simulink model "plant"  (R2020a)
settings: Solver=VariableStepAuto  StartTime=0.0  StopTime=20.0  RelTol=1e-3
values from neighbouring files (symbols this model uses):
  Ts = 0.1    [main_adaptive_mpc.m]
libraries: sharedtransform x1, shared6dof x1, mpclib x1
settings Model: Creator=Lamarre  LastModifiedBy=Lamarre

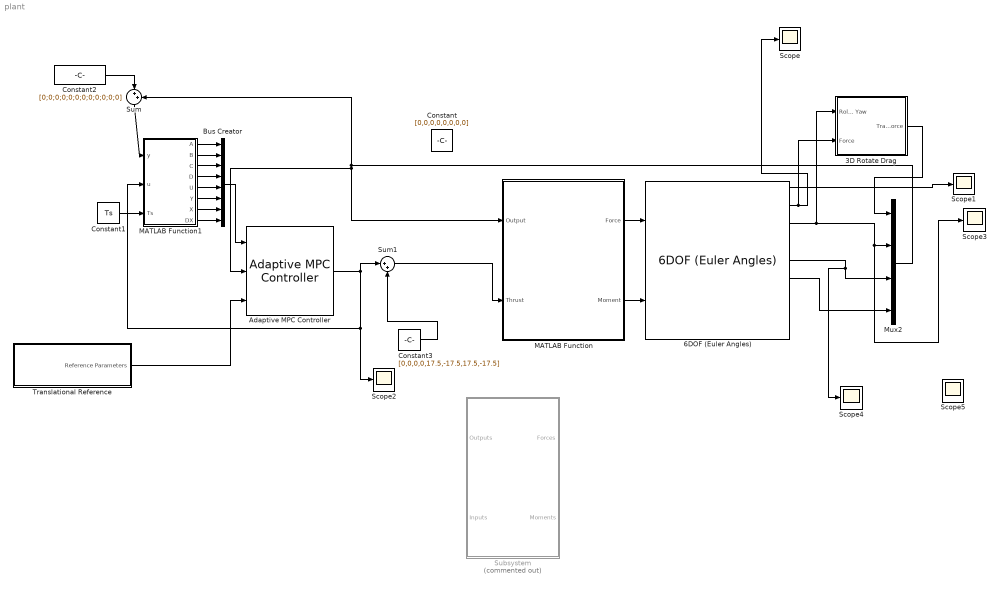
== system plant ==
  3D Rotate Drag : Subsystem
  6DOF (Euler Angles) : shared6dof/6DOF (Euler Angles)  units=Metric (MKS)  mtype=Fixed  rep=Euler Angles  xme_0=[0 0 0]  Vm_0=[0 0 0]  eul_0=[0 0 0]  pm_0=[0 0 0]  mass_0=mass  mass_e=0.5  mass_f=2.0  inertia=I  inertia_e=eye(3)  inertia_f=2*eye(3)  k_quat=1.0  vre_flag=on  abi_flag=on  aMode=0  xme_statename=''  Vm_statename=''  eul_statename=''  quat_statename=''  pm_statename=''  mass_statename=''
      settings: SourceProductBaseCode=AE,PW,MT,VE,VP
  Adaptive MPC Controller : mpclib/Adaptive MPC Controller  SCDEnableBlockLinearizationSpecification=on  mpcobj=mpcobj  enable_value=0  updateMPCinCallerWorkspace=on  md_inport=off  mv_inport=off  uref_inport=off  return_cost=off  return_mvseq=off  return_qpstatus=off  return_xseq=off  return_state=off  return_ovseq=off  state_inport=off  isltv_plant=off  umin_inport=off  umax_inport=off  ymin_inport=off  ymax_inport=off  cc_inport=off  ywt_inport=off  uwt_inport=off  duwt_inport=off  rhoeps_inport=off  pm_inport=off  MaximumP=10  HorizonChoice=FixedHorizon  BlockDataType=double  SampleTimeInherited=off  switch_inport=off
  Bus Creator : BusCreator  Inputs=8
  Constant : Constant  Value=[0,0,0,0,0,0,0,0]
  Constant1 : Constant  Value=Ts
  Constant2 : Constant  Value=[0;0;0;0;0;0;0;0;0;0;0;0]  VectorParams1D=off
  Constant3 : Constant  Value=[0,0,0,0,17.5,-17.5,17.5,-17.5]
  MATLAB Function : MATLAB Function  TreatAsAtomicUnit=on
  MATLAB Function1 : MATLAB Function  TreatAsAtomicUnit=on
  Mux2 : Mux
  Scope{,1..5} (6 alike) : Scope
  Subsystem : Subsystem  Commented=on
  Sum : Sum  Inputs=|++
  Sum1 : Sum  Inputs=|++
  Translational Reference : Subsystem
  wires:
  6DOF (Euler Angles)/3 -> Scope3/1, Mux2/2, 3D Rotate Drag/1("Roll, Pitch, Yaw")
  6DOF (Euler Angles)/5 -> Scope4/1, Mux2/3
  6DOF (Euler Angles)/6 -> Mux2/4
  Mux2/1 -> MATLAB Function/1(Output), Adaptive MPC Controller/2, Sum/2
  Adaptive MPC Controller/1 -> Scope2/1, MATLAB Function1/2(u), Sum1/1
  MATLAB Function1/4(D) -> Bus Creator/4
  MATLAB Function1/1(A) -> Bus Creator/1
  MATLAB Function1/6(Y) -> Bus Creator/6
  MATLAB Function1/2(B) -> Bus Creator/2
  MATLAB Function1/5(U) -> Bus Creator/5
  MATLAB Function1/7(X) -> Bus Creator/7
  MATLAB Function1/8(DX) -> Bus Creator/8
  MATLAB Function1/3(C) -> Bus Creator/3
  Bus Creator/1 -> Adaptive MPC Controller/1
  Translational Reference/1(Reference Parameters) -> Adaptive MPC Controller/3
  Constant1/1 -> MATLAB Function1/3(Ts)
  Constant2/1 -> Sum/1
  Sum/1 -> MATLAB Function1/1(y)
  6DOF (Euler Angles)/1 -> Scope1/1
  6DOF (Euler Angles)/2 -> 3D Rotate Drag/2(Force), Scope/1
  3D Rotate Drag/1("Transformed_Force ") -> Mux2/1
  Constant3/1 -> Sum1/2
  MATLAB Function/1(Force) -> 6DOF (Euler Angles)/1
  MATLAB Function/2(Moment) -> 6DOF (Euler Angles)/2
  Sum1/1 -> MATLAB Function/2(Thrust)

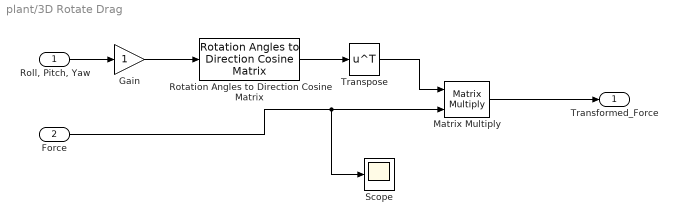
== system plant/3D Rotate Drag ==
  "Roll, Pitch, Yaw" : Inport
  Force : Inport  Port=2
  Gain : Gain
  Matrix Multiply : Product  Multiplication=Matrix(*)
  Rotation Angles to Direction Cosine Matrix : sharedtransform/Rotation Angles to Direction Cosine Matrix  rotationOrder=XYZ  aMode=aMode
      settings: SourceProductBaseCode=AE,PW,MT,VE,VP
  Scope : Scope
  Transpose : Math  Operator=transpose  SignedPower=on  SaturateOnIntegerOverflow=on
  "Transformed_Force " : Outport  VectorParamsAs1DForOutWhenUnconnected=off
  wires:
  Matrix Multiply/1 -> "Transformed_Force "/1
  Rotation Angles to Direction Cosine Matrix/1 -> Transpose/1
  Force/1 -> Scope/1, Matrix Multiply/2
  "Roll, Pitch, Yaw"/1 -> Gain/1
  Transpose/1 -> Matrix Multiply/1
  Gain/1 -> Rotation Angles to Direction Cosine Matrix/1

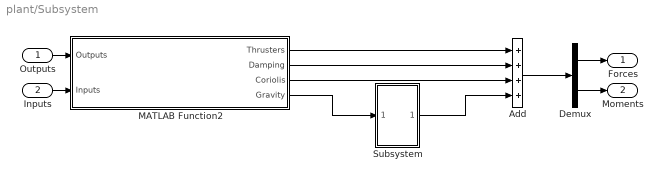
== system plant/Subsystem ==
  Outputs : Inport
  Inputs : Inport  Port=2
  Add : Sum  Inputs=++++
  Demux : Demux  Outputs=2
  MATLAB Function2 : MATLAB Function  TreatAsAtomicUnit=on
  Subsystem : Subsystem
  Forces : Outport
  Moments : Outport  Port=2
  wires:
  Inputs/1 -> MATLAB Function2/2(Inputs)
  Outputs/1 -> MATLAB Function2/1(Outputs)
  MATLAB Function2/3(Coriolis) -> Add/3
  MATLAB Function2/2(Damping) -> Add/2
  MATLAB Function2/1(Thrusters) -> Add/1
  Add/1 -> Demux/1
  Demux/1 -> Forces/1
  Demux/2 -> Moments/1
  MATLAB Function2/4(Gravity) -> Subsystem/1(In1)
  Subsystem/1(Out1) -> Add/4

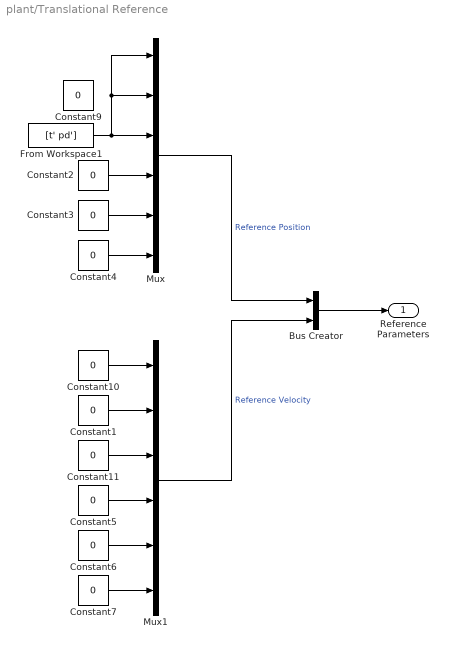
== system plant/Translational Reference ==
  Bus Creator : BusCreator  Inputs=2
  Constant{1..7,9..11} (10 alike) : Constant  Value=0
  From Workspace1 : FromWorkspace  VariableName=[t' pd']
  Mux : Mux  Inputs=6
  Mux1 : Mux  Inputs=6
  Reference Parameters : Outport  VectorParamsAs1DForOutWhenUnconnected=off
  wires:
  Mux/1 -> Bus Creator/1  "Reference Position"
  Mux1/1 -> Bus Creator/2  "Reference Velocity"
  Bus Creator/1 -> Reference Parameters/1
  Constant1/1 -> Mux1/2
  Constant2/1 -> Mux/4
  Constant3/1 -> Mux/5
  Constant4/1 -> Mux/6
  Constant6/1 -> Mux1/5
  Constant7/1 -> Mux1/6
  Constant5/1 -> Mux1/4
  Constant10/1 -> Mux1/1
  Constant11/1 -> Mux1/3
  From Workspace1/1 -> Mux/2, Mux/1, Mux/3

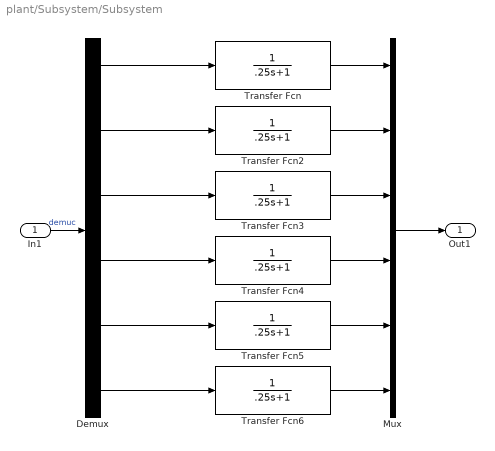
== system plant/Subsystem/Subsystem ==
  In1 : Inport
  Demux : Demux  Outputs=6
  Mux : Mux  Inputs=6
  Transfer Fcn{,2..6} (6 alike) : TransferFcn  Denominator=[.25 1]
  Out1 : Outport
  wires:
  Demux/1 -> Transfer Fcn/1
  In1/1 -> Demux/1  "demuc"
  Demux/2 -> Transfer Fcn2/1
  Demux/3 -> Transfer Fcn3/1
  Demux/4 -> Transfer Fcn4/1
  Demux/5 -> Transfer Fcn5/1
  Demux/6 -> Transfer Fcn6/1
  Transfer Fcn/1 -> Mux/1
  Transfer Fcn2/1 -> Mux/2
  Transfer Fcn3/1 -> Mux/3
  Transfer Fcn4/1 -> Mux/4
  Transfer Fcn5/1 -> Mux/5
  Transfer Fcn6/1 -> Mux/6
  Mux/1 -> Out1/1

== matlab function plant/MATLAB Function ==
  data: Output input; Force output; Thrust input; Moment output
function [Force,Moment] = Calculate_Forces_and_Torques(Output,Thrust)
Dynamics=AUVForceMoments(Output,Thrust);
Force=Dynamics(1:3);
Moment= Dynamics(4:6);

== matlab function plant/Subsystem/MATLAB Function2 ==
  data: Outputs input; Thrusters output; Inputs input; Damping output; Coriolis output; Gravity output
function [Thrusters,Damping,Coriolis,Gravity] = Calculate_AUV_Dynamics(Outputs,Inputs)
Dynamics=AUVDynamics(Outputs,Inputs);

Thrusters= Dynamics(1:6);
Damping=Dynamics(7:12);
Coriolis=Dynamics(13:18);
Gravity= Dynamics(19:24);

== matlab function plant/MATLAB Function1 ==
  data: y input; u input; A output; Ts input; B output; C output; D output; U output; Y output; X output; DX output
function [A,B,C,D,U,Y,X,DX] = Plant(y,u,Ts)
% Lineariser le model dynamique

%x=[y(4:5,1);y(7:12,1)];
%x(5)=x(5)-.85;
[Ac, Bc, Cc, Dc]=AUVStateJacobianFcn(y,u);
% Generate discrete-time model

%  nx = size(Ac,1);
%  nu = size(Bc,2);
%cplant=ss(Ac,Bc,Cc,Dc);
%plant=c2d(cplant,Ts,'zoh');

nx = size(Ac,1);
nu = size(Bc,2);
M = expm([[Ac Bc]*Ts; zeros(nu,nu+nx)]);
A = M(1:nx,1:nx);
B = M(1:nx,nx+1:nx+nu);
C = Cc;
D = Dc;
 %xx=[X(4:5,1);X(7:12)];

% cplant=ss(Ac,Bc,Cc,Dc);
% plant=c2d(cplant,Ts,'zoh');
%plant=ss(A,B,C,D,Ts);

% Nominal conditions for discrete-time plant
U=u.';
Y=(Cc*y + Dc*u).';
X=y.';
DX=(A*y+B*u-y).';
